simulink library "jud"  (Simulink 8.1)
settings: Solver=ode45  StartTime=0.0  StopTime=10.0  RelTol=1e-3
libraries: jcc x1, jcw x1, jeb x1
settings Model: Creator=xsellart  LastModifiedBy=AT015555

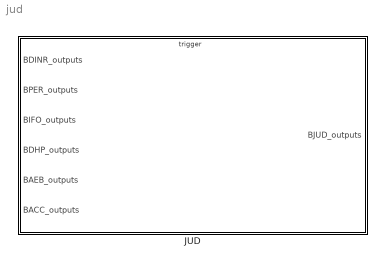
== system jud ==
  JUD : Subsystem

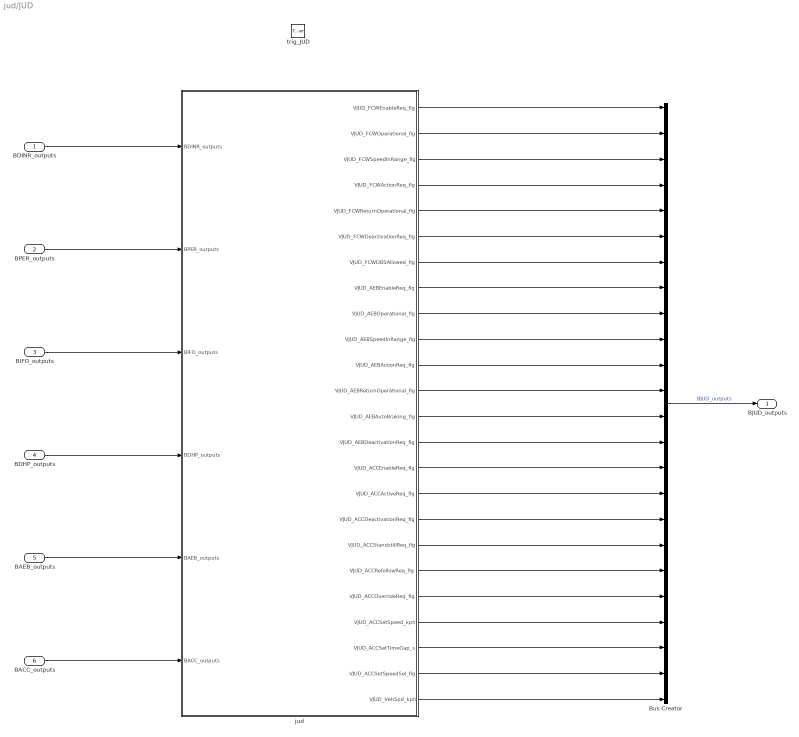
== system jud/JUD ==
  BDINR_outputs : Inport  OutDataTypeStr=Bus: BDINR_outputs
  BPER_outputs : Inport  Port=2  OutDataTypeStr=Bus: BPER_outputs
  BIFO_outputs : Inport  Port=3  OutDataTypeStr=Bus: BIFO_outputs
  BDHP_outputs : Inport  Port=4  OutDataTypeStr=Bus: BDHP_outputs
  BAEB_outputs : Inport  Port=5  OutDataTypeStr=Bus: BAEB_outputs
  BACC_outputs : Inport  Port=6  OutDataTypeStr=Bus: BACC_outputs
  trig_JUD : TriggerPort  TriggerType=function-call
      settings: AttributesFormatString=State = %<StatesWhenEnabling>
  Bus Creator : BusCreator  Inputs=24  OutDataTypeStr=Bus: BJUD_outputs
  jud : Subsystem
  BJUD_outputs : Outport  OutDataTypeStr=Bus: BJUD_outputs
  wires:
  jud/24(VJUD_VehSpd_kph) -> Bus Creator/24
  jud/20(VJUD_ACCOverrideReq_flg) -> Bus Creator/20
  jud/5(VJUD_FCWReturnOperational_flg) -> Bus Creator/5
  jud/6(VJUD_FCWDeactivationReq_flg) -> Bus Creator/6
  jud/19(VJUD_ACCRefollowReq_flg) -> Bus Creator/19
  jud/21(VJUD_ACCSetSpeed_kph) -> Bus Creator/21
  jud/18(VJUD_ACCStandstillReq_flg) -> Bus Creator/18
  jud/1(VJUD_FCWEnableReq_flg) -> Bus Creator/1
  jud/2(VJUD_FCWOperational_flg) -> Bus Creator/2
  jud/22(VJUD_ACCSetTimeGap_s) -> Bus Creator/22
  jud/9(VJUD_AEBOperational_flg) -> Bus Creator/9
  jud/15(VJUD_ACCEnableReq_flg) -> Bus Creator/15
  jud/13(VJUD_AEBAutoBraking_flg) -> Bus Creator/13
  jud/14(VJUD_AEBDeactivationReq_flg) -> Bus Creator/14
  jud/3(VJUD_FCWSpeedInRange_flg) -> Bus Creator/3
  jud/16(VJUD_ACCActiveReq_flg) -> Bus Creator/16
  jud/8(VJUD_AEBEnableReq_flg) -> Bus Creator/8
  jud/4(VJUD_FCWActionReq_flg) -> Bus Creator/4
  jud/17(VJUD_ACCDeactivationReq_flg) -> Bus Creator/17
  jud/11(VJUD_AEBActionReq_flg) -> Bus Creator/11
  jud/7(VJUD_FCWDBSAllowed_flg) -> Bus Creator/7
  jud/10(VJUD_AEBSpeedInRange_flg) -> Bus Creator/10
  jud/23(VJUD_ACCSetSpeedSel_flg) -> Bus Creator/23
  jud/12(VJUD_AEBReturnOperational_flg) -> Bus Creator/12
  Bus Creator/1 -> BJUD_outputs/1  "BJUD_outputs"
  BDINR_outputs/1 -> jud/1(BDINR_outputs)
  BPER_outputs/1 -> jud/2(BPER_outputs)
  BIFO_outputs/1 -> jud/3(BIFO_outputs)
  BDHP_outputs/1 -> jud/4(BDHP_outputs)
  BAEB_outputs/1 -> jud/5(BAEB_outputs)
  BACC_outputs/1 -> jud/6(BACC_outputs)

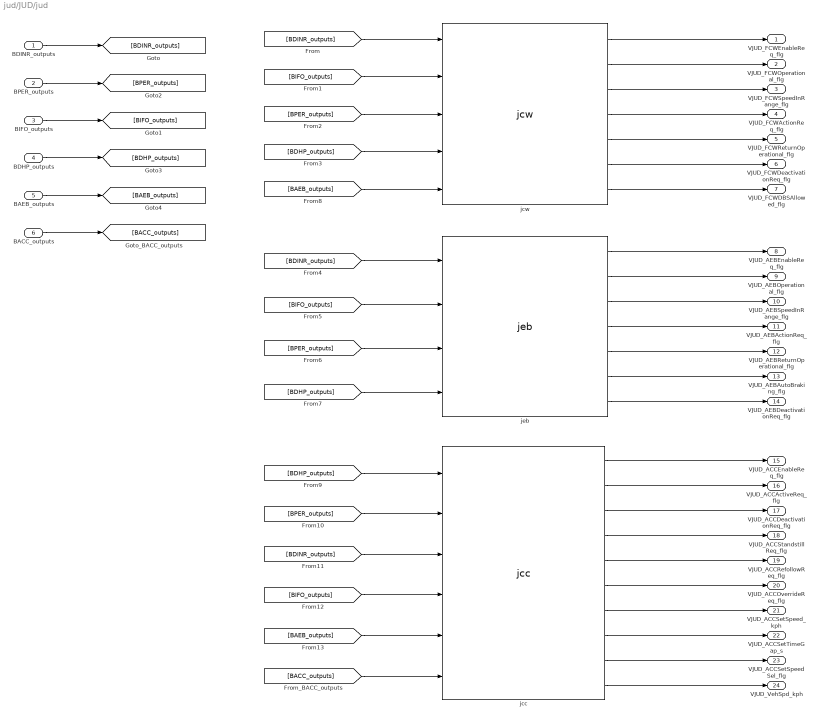
== system jud/JUD/jud ==
  BDINR_outputs : Inport  OutDataTypeStr=Bus: BDINR_outputs
  BPER_outputs : Inport  Port=2  OutDataTypeStr=Bus: BPER_outputs
  BIFO_outputs : Inport  Port=3  OutDataTypeStr=Bus: BIFO_outputs
  BDHP_outputs : Inport  Port=4  OutDataTypeStr=Bus: BDHP_outputs
  BAEB_outputs : Inport  Port=5  OutDataTypeStr=Bus: BAEB_outputs
  BACC_outputs : Inport  Port=6  OutDataTypeStr=Bus: BACC_outputs
  jcc : jcc/jcc
  jcw : jcw/jcw
  jeb : jeb/jeb
  VJUD_FCWEnableReq_flg : Outport
  VJUD_FCWOperational_flg : Outport  Port=2
  VJUD_FCWSpeedInRange_flg : Outport  Port=3
  VJUD_FCWActionReq_flg : Outport  Port=4
  VJUD_FCWReturnOperational_flg : Outport  Port=5
  VJUD_FCWDeactivationReq_flg : Outport  Port=6
  VJUD_FCWDBSAllowed_flg : Outport  Port=7
  VJUD_AEBEnableReq_flg : Outport  Port=8
  VJUD_AEBOperational_flg : Outport  Port=9
  VJUD_AEBSpeedInRange_flg : Outport  Port=10
  VJUD_AEBActionReq_flg : Outport  Port=11
  VJUD_AEBReturnOperational_flg : Outport  Port=12
  VJUD_AEBAutoBraking_flg : Outport  Port=13
  VJUD_AEBDeactivationReq_flg : Outport  Port=14
  VJUD_ACCEnableReq_flg : Outport  Port=15
  VJUD_ACCActiveReq_flg : Outport  Port=16
  VJUD_ACCDeactivationReq_flg : Outport  Port=17
  VJUD_ACCStandstillReq_flg : Outport  Port=18
  VJUD_ACCRefollowReq_flg : Outport  Port=19
  VJUD_ACCOverrideReq_flg : Outport  Port=20
  VJUD_ACCSetSpeed_kph : Outport  Port=21
  VJUD_ACCSetTimeGap_s : Outport  Port=22
  VJUD_ACCSetSpeedSel_flg : Outport  Port=23
  VJUD_VehSpd_kph : Outport  Port=24
  wires:
  jcc/10 -> VJUD_VehSpd_kph/1
  [BIFO_outputs] -> jcw/2
  jeb/1 -> VJUD_AEBEnableReq_flg/1
  [BPER_outputs] -> jcw/3
  jcw/1 -> VJUD_FCWEnableReq_flg/1
  jcw/7 -> VJUD_FCWDBSAllowed_flg/1
  [BIFO_outputs] -> jeb/2
  [BDINR_outputs] -> jeb/1
  BPER_outputs/1 -> [BPER_outputs]
  jcw/6 -> VJUD_FCWDeactivationReq_flg/1
  jeb/6 -> VJUD_AEBAutoBraking_flg/1
  BIFO_outputs/1 -> [BIFO_outputs]
  BDHP_outputs/1 -> [BDHP_outputs]
  jcw/4 -> VJUD_FCWActionReq_flg/1
  [BDHP_outputs] -> jcw/4
  jcw/2 -> VJUD_FCWOperational_flg/1
  [BDHP_outputs] -> jeb/4
  jcw/3 -> VJUD_FCWSpeedInRange_flg/1
  jeb/4 -> VJUD_AEBActionReq_flg/1
  [BDINR_outputs] -> jcw/1
  [BPER_outputs] -> jeb/3
  BDINR_outputs/1 -> [BDINR_outputs]
  jeb/7 -> VJUD_AEBDeactivationReq_flg/1
  BAEB_outputs/1 -> [BAEB_outputs]
  [BAEB_outputs] -> jcw/5
  jeb/2 -> VJUD_AEBOperational_flg/1
  jeb/3 -> VJUD_AEBSpeedInRange_flg/1
  jcw/5 -> VJUD_FCWReturnOperational_flg/1
  jeb/5 -> VJUD_AEBReturnOperational_flg/1
  jcc/2 -> VJUD_ACCActiveReq_flg/1
  jcc/3 -> VJUD_ACCDeactivationReq_flg/1
  jcc/1 -> VJUD_ACCEnableReq_flg/1
  jcc/4 -> VJUD_ACCStandstillReq_flg/1
  jcc/5 -> VJUD_ACCRefollowReq_flg/1
  jcc/6 -> VJUD_ACCOverrideReq_flg/1
  jcc/7 -> VJUD_ACCSetSpeed_kph/1
  jcc/8 -> VJUD_ACCSetTimeGap_s/1
  jcc/9 -> VJUD_ACCSetSpeedSel_flg/1
  [BDHP_outputs] -> jcc/1
  [BPER_outputs] -> jcc/2
  [BDINR_outputs] -> jcc/3
  [BIFO_outputs] -> jcc/4
  [BAEB_outputs] -> jcc/5
  BACC_outputs/1 -> [BACC_outputs]
  [BACC_outputs] -> jcc/6
